simulink model "lab1"  (R2024a)
settings: Solver=VariableStepAuto  StartTime=0.0  StopTime=50  RelTol=1e-3
libraries: simulink x1
settings Model: Creator=psp_dada  LastModifiedBy=psp_dada

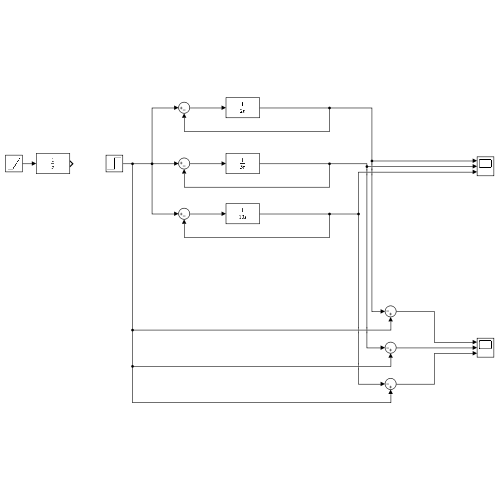
[thumbnail: Simulink's stored preview of the top-level diagram]
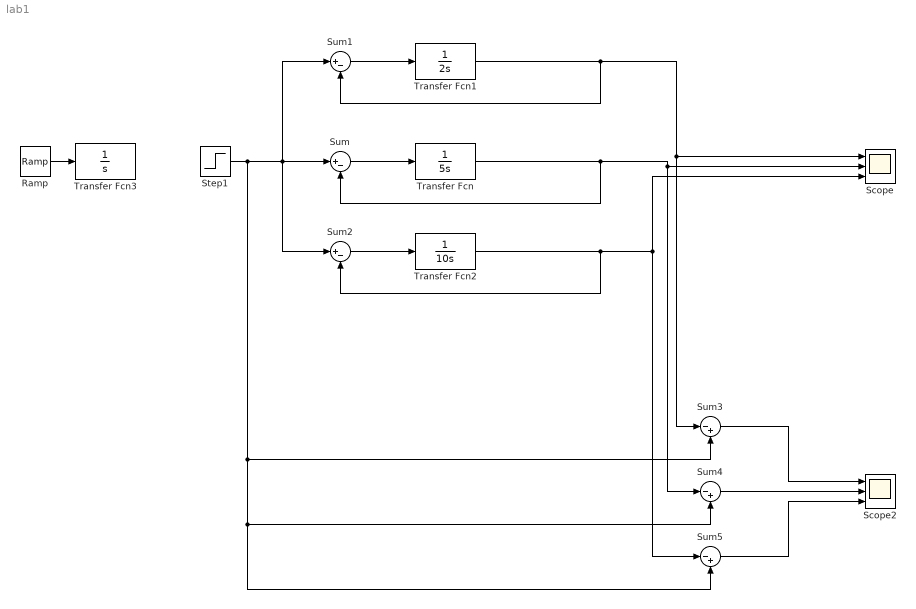
== system lab1 ==
  Ramp : simulink/Sources/Ramp  slope=1  start=0  InitialOutput=0
  Scope : Scope  NumInputPorts=3
  Scope2 : Scope  NumInputPorts=3
  Step1 : Step  SampleTime=0
  Sum : Sum  Inputs=|+-
  Sum1 : Sum  Inputs=|+-
  Sum2 : Sum  Inputs=|+-
  Sum3 : Sum  Inputs=|-+
  Sum4 : Sum  Inputs=|-+
  Sum5 : Sum  Inputs=|-+
  Transfer Fcn : TransferFcn  Denominator=[5 0]
  Transfer Fcn1 : TransferFcn  Denominator=[2 0]  ContinuousStateAttributes='aaa'
  Transfer Fcn2 : TransferFcn  Denominator=[10 0]
  Transfer Fcn3 : TransferFcn  Denominator=[1 0]  ContinuousStateAttributes='aaa'
  wires:
  Sum/1 -> Transfer Fcn/1
  Transfer Fcn/1 -> Sum/2, Scope/2, Sum4/1
  Transfer Fcn1/1 -> Sum1/2, Scope/1, Sum3/1
  Sum1/1 -> Transfer Fcn1/1
  Transfer Fcn2/1 -> Scope/3, Sum5/1, Sum2/2
  Sum2/1 -> Transfer Fcn2/1
  Step1/1 -> Sum2/1, Sum1/1, Sum/1, Sum5/2, Sum4/2, Sum3/2
  Sum3/1 -> Scope2/1
  Sum4/1 -> Scope2/2
  Sum5/1 -> Scope2/3
  Ramp/1 -> Transfer Fcn3/1
